simulink model "KUKA_KR10_R1100_ROS"  (R2024a)
settings: Solver=ode15s  StartTime=0.0  StopTime=6  RelTol=1e-9  AbsTol=1e-9  EnableMultiTasking=on
model workspace (MAT data in the model file):
  XSize = 1
values from neighbouring files (symbols this model uses):
  dichte_alu = 2700    [Parameter.m]    (also in workspace_test.mat)
  N = length(accelX)    [pds.m]
undefined symbols (not defined in the file or in its folder): th_J1, th_J2, th_J3, th_J4, th_J5, th_J6, th_transition_factor, X, Y, Z
libraries: sm_lib x70, nesl_utility x30
(part 1 of 3)
settings Model: Creator=beth0005  LastModifiedBy=Johannes
settings SolverCC: AutoScaleAbsTol=off  AlgebraicLoopSolver=TrustRegion
settings DataIOCC: LimitDataPoints=on  MaxDataPoints=10000
settings OptimizationCC: LifeSpan=inf
settings DebuggingCC: UnconnectedInputMsg=warning  UnconnectedOutputMsg=warning  UnconnectedLineMsg=warning  AllowSymbolicDim=off  SFUnexpectedBacktrackingDiag=warning  SFNoUnconditionalDefaultTransitionDiag=warning  SFExecutionAtInitializationDiag=none  ArithmeticOperatorsInVariantConditions=warning
settings ModelReferenceCC: EnableRefExpFcnMdlSchedulingChecks=on
settings SFSimCC: SimUseLocalCustomCode=off  CustomCodeUndefinedFunction=UseInterfaceOnly
settings RTWCC: RTWUseLocalCustomCode=off  GPUComputeCapability=3.5  DLArmComputeVersion=19.05
settings CodeAppCC: StateflowObjectComments=on
settings GRTTargetCC: TargetLangStandard=C89/C90 (ANSI)
settings ConfigComp: CovMetricSettings=dw  CovSaveCumulativeToWorkspaceVar=on  CovSaveSingleToWorkspaceVar=on  CovExternalEMLEnable=off  CovSFcnEnable=off
settings SimscapeCC: SimscapeLogType=all  SimscapeLogSimulationStatistics=on  SimscapeLogDataHistory=10000

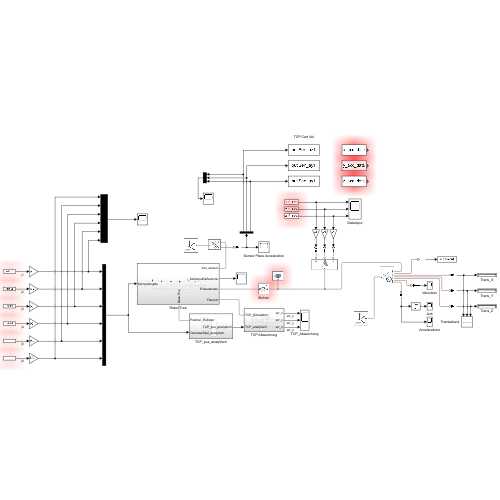
[thumbnail: Simulink's stored preview of the top-level diagram]
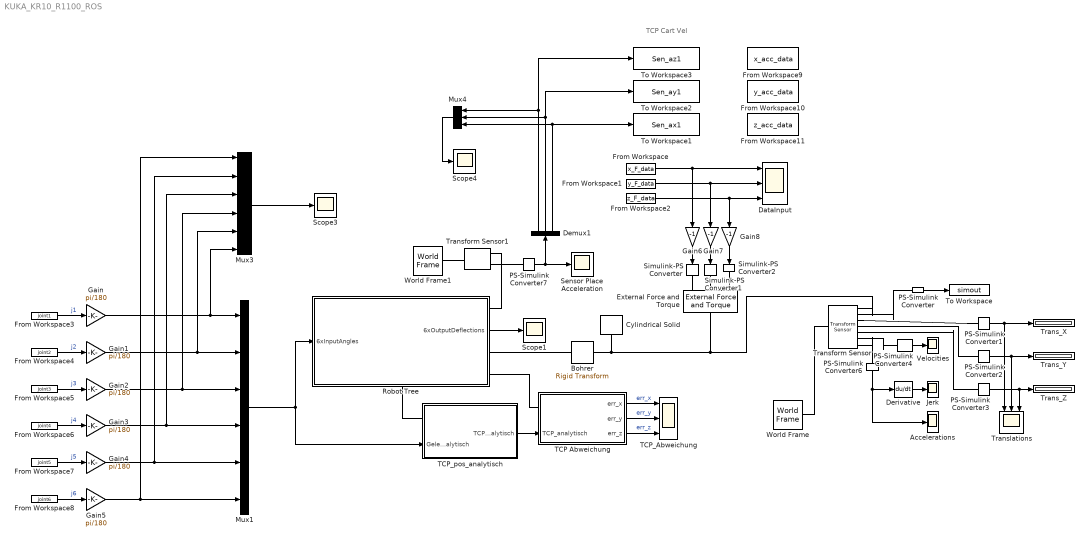
== system KUKA_KR10_R1100_ROS ==
  note: TCP Cart Vel
  Accelerations : Scope
  Bohrer : sm_lib/Frames and Transforms/Rigid Transform  RotationMethod=None  FollAlignAxisA=+X  BaseAlignAxisA=+Y  FollAlignAxisB=+Y  BaseAlignAxisB=+Z  RotationStandardAxis=+Y  RotationAngle=90  RotationAngleUnits=deg  RotationArbitraryAxis=[0 0 1]  RotationSequenceAxes=FollowerAxes  RotationSequence=XYX  RotationSequenceAngles=[0 0 0]  RotationSequenceAnglesUnits=deg  RotationMatrix=[1 0 0; 0 1 0; 0 0 1]  Quaternion=[1 0 0 0]  TranslationMethod=StandardAxis  TranslationCartesianOffset=[0 0 63]  TranslationCartesianOffsetUnits=mm  TranslationStandardAxis=+Z  TranslationStandardOffset=lang_bohrer  TranslationStandardOffsetUnits=mm  TranslationROffset=0  TranslationROffsetUnits=m  TranslationThetaOffset=0  TranslationThetaOffsetUnits=deg  TranslationZOffset=0  TranslationZOffsetUnits=m
  Cylindrical Solid : sm_lib/Body Elements/Cylindrical Solid  CylinderRadius=4  CylinderRadiusUnits=mm  CylinderLength=63  CylinderLengthUnits=mm  ExportEntireGeometry=off  InertiaType=CalculateFromGeometry  BasedOnType=Density  Density=dichte_alu  DensityUnits=kg/m^3  Mass=1  MassUnits=kg  CenterOfMass=[0 0 0]  CenterOfMassUnits=m  MomentsOfInertia=[1 1 1]  MomentsOfInertiaUnits=kg*m^2  ProductsOfInertia=[0 0 0]  ProductsOfInertiaUnits=kg*m^2  GraphicType=FromGeometry  MarkerShape=Sphere  MarkerSize=10  GraphicVisPropType=SimpleVisualProperties  GraphicDiffuseColor=[0.5 0.5 0.5]  GraphicOpacity=1  GraphicSpecularColor=[0.5 0.5 0.5 1.0]  GraphicAmbientColor=[0.15 0.15 0.15 1.0]  GraphicEmissiveColor=[0.0 0.0 0.0 1.0]  GraphicShininess=75  DoExposeReferenceFrame=off  SerializedFrames=<Frames><Frame><Id>Frame1</Id><Value><Name>F1</Name><Origin><Source>GeometricFeature</Source><FeatureName>top surface</FeatureName></Origin><PrimaryAxis><DefinedDirection>+Z</DefinedDirection><Source>ReferenceFrame</Source><SourceDirection>+Z</SourceDirection><FeatureName></FeatureName></PrimaryAxis><SecondaryAxis><DefinedDirection>+X</DefinedDirection><Source>ReferenceFrame</Source><SourceDirection>+X</SourceDirection><FeatureName></FeatureName></SecondaryAxis></Value></Frame></Frames>
  DataInput : Scope  NumInputPorts=3
  Demux1 : Demux  Outputs=3
  Derivative : Derivative
  External Force and Torque : sm_lib/Forces and Torques/External Force and Torque  EnableForceX=on  EnableForceY=on  EnableForceZ=on  EnableForce=off  ForceResolutionFrame=AttachedFrame  EnableTorqueX=off  EnableTorqueY=off  EnableTorqueZ=off  EnableTorque=off  TorqueResolutionFrame=AttachedFrame
  From Workspace : FromWorkspace  VariableName=x_F_data  SampleTime=-1
  From Workspace1 : FromWorkspace  VariableName=y_F_data  SampleTime=-1
  From Workspace10 : FromWorkspace  VariableName=y_acc_data  SampleTime=-1
  From Workspace11 : FromWorkspace  VariableName=z_acc_data  SampleTime=-1
  From Workspace2 : FromWorkspace  VariableName=z_F_data  SampleTime=-1
  From Workspace3 : FromWorkspace  VariableName=joint1  SampleTime=-1
  From Workspace4 : FromWorkspace  VariableName=joint2  SampleTime=-1
  From Workspace5 : FromWorkspace  VariableName=joint3  SampleTime=-1
  From Workspace6 : FromWorkspace  VariableName=joint4  SampleTime=-1
  From Workspace7 : FromWorkspace  VariableName=joint5  SampleTime=-1
  From Workspace8 : FromWorkspace  VariableName=joint6  SampleTime=-1
  From Workspace9 : FromWorkspace  VariableName=x_acc_data  SampleTime=-1
  Gain{,1..5} (6 alike) : Gain  Gain=pi/180
  Gain6 : Gain  Gain=-1
  Gain7 : Gain  Gain=-1
  Gain8 : Gain  Gain=-1
  Jerk : Scope
  Mux1 : Mux  Inputs=6
  Mux3 : Mux  Inputs=6
  Mux4 : Mux  Inputs=3
  PS-Simulink Converter{,1..4,6..7} (7 alike) : nesl_utility/PS-Simulink Converter  PhysicalDomain=network_engine_domain  SubClassName=ps_output  LeftPortType=input  RightPortType=output  PseudoPeriodic=off  Frequencies=[]  VectorFormat=inherit  Unit=inherit  AffineConversion=off
  Robot Tree : Subsystem
      settings: PortSchema="{\"entries\":[{\"content\":{\"sides\":[{\"content\":{\"connectorIds\":[\"In1\"]},\"type\":\"ConnectorPlacement.EquallySpacedRectSide\",\"uuid\":\"83afddbe-1d35-4f48-9dd2-c5eddaf741d9\"},{\"content\":{\"connectorIds\":[\"RConn1\",\"Out1\",\"RConn2\",\"RConn3\"],\"side\":\"RIGHT\"},\"type\":\"ConnectorPlacement.EquallySpacedRectSide\",\"uuid\":\"b2a35604-11db-400a-b921-df56b5b1bdc7\"},{\"content\":{\"side\":\"TOP\"},\"type\":\"ConnectorPlacement.EquallySpacedRectSide\",\"uuid\":\"d988bacb-7459-4110-a132-4d0586d8e44f\"},{\"content\":{\"connectorIds\":[\"RConn4\"],\"side\":\"BOTTOM\"},\"type\":\"ConnectorPlacement.EquallySpacedRectSide\",\"uuid\":\"784d5e4a-8f9a-40d1-a5c6-3fcb642770f1\"}]},\"type\":\"ConnectorPlacement.EquallySpacedConnector\",\"uuid\":\"99878518-e7fe-4a6a-9eb0-094d259cda0e\"}],\"packageUris\":[\"http://schema.mathworks.com/mf0/Connector/R2020b\"],\"version\":\"1.0\"}"
  Scope1 : Scope
  Scope3 : Scope
  Scope4 : Scope
  Sensor Place Acceleration : Scope
  Simulink-PS Converter : nesl_utility/Simulink-PS Converter  PhysicalDomain=network_engine_domain  SubClassName=ps_input  LeftPortType=input  RightPortType=output  PseudoPeriodic=off  Frequencies=[]  NoiseDistribution=none  NoiseParameters=[]  Unit=1  AffineConversion=off  FilteringAndDerivatives=filter  SimscapeFilterOrder=2  InputFilterTimeConstant=0.0001  UdotUserProvided=0
  Simulink-PS Converter1 : nesl_utility/Simulink-PS Converter  PhysicalDomain=network_engine_domain  SubClassName=ps_input  LeftPortType=input  RightPortType=output  PseudoPeriodic=off  Frequencies=[]  NoiseDistribution=none  NoiseParameters=[]  Unit=1  AffineConversion=off  FilteringAndDerivatives=filter  SimscapeFilterOrder=2  InputFilterTimeConstant=0.0001  UdotUserProvided=0
  Simulink-PS Converter2 : nesl_utility/Simulink-PS Converter  PhysicalDomain=network_engine_domain  SubClassName=ps_input  LeftPortType=input  RightPortType=output  PseudoPeriodic=off  Frequencies=[]  NoiseDistribution=none  NoiseParameters=[]  Unit=1  AffineConversion=off  FilteringAndDerivatives=filter  SimscapeFilterOrder=2  InputFilterTimeConstant=0.0001  UdotUserProvided=0
  TCP Abweichung : Subsystem
      settings: PortSchema="{\"entries\":[{\"content\":{\"sides\":[{\"content\":{\"connectorIds\":[\"LConn1\",\"In1\"]},\"type\":\"ConnectorPlacement.EquallySpacedRectSide\",\"uuid\":\"8fbb3f34-d7d1-4090-9281-a387436a6191\"},{\"content\":{\"connectorIds\":[\"Out1\",\"Out2\",\"Out3\"],\"side\":\"RIGHT\"},\"type\":\"ConnectorPlacement.EquallySpacedRectSide\",\"uuid\":\"2461bf91-e690-4063-84b2-ad7cc9454b37\"},{\"content\":{\"side\":\"TOP\"},\"type\":\"ConnectorPlacement.EquallySpacedRectSide\",\"uuid\":\"0fbb9cfb-49b2-42f2-b0a5-a9e967349aea\"}]},\"type\":\"ConnectorPlacement.EquallySpacedConnector\",\"uuid\":\"5e1e4f46-aaa2-4a76-a14e-db38171314b7\"}],\"packageUris\":[\"http://schema.mathworks.com/mf0/Connector/R2020b\"],\"version\":\"1.0\"}"
  TCP_Abweichung : Scope  NumInputPorts=3
  TCP_pos_analytisch : Subsystem
      settings: PortSchema="{\"entries\":[{\"content\":{\"sides\":[{\"content\":{\"connectorIds\":[\"LConn1\",\"In1\"]},\"type\":\"ConnectorPlacement.EquallySpacedRectSide\",\"uuid\":\"538ee7b4-053d-4344-bb82-6fadd6800804\"},{\"content\":{\"connectorIds\":[\"Out1\"],\"side\":\"RIGHT\"},\"type\":\"ConnectorPlacement.EquallySpacedRectSide\",\"uuid\":\"6da0b3fa-3dd3-4693-bc25-55cdb306fc09\"},{\"content\":{\"side\":\"TOP\"},\"type\":\"ConnectorPlacement.EquallySpacedRectSide\",\"uuid\":\"c57a0aac-3147-45b1-888e-d3700a099c5d\"}]},\"type\":\"ConnectorPlacement.EquallySpacedConnector\",\"uuid\":\"ef060d6a-5fd8-4986-b270-7bf484a81e58\"}],\"packageUris\":[\"http://schema.mathworks.com/mf0/Connector/R2020b\"],\"version\":\"1.0\"}"
  To Workspace : ToWorkspace  VariableName=simout  SaveFormat=Structure  SampleTime=-1
  To Workspace1 : ToWorkspace  VariableName=Sen_ax1  SaveFormat=Timeseries  SampleTime=-1
  To Workspace2 : ToWorkspace  VariableName=Sen_ay1  SaveFormat=Timeseries  SampleTime=-1
  To Workspace3 : ToWorkspace  VariableName=Sen_az1  SaveFormat=Timeseries  SampleTime=-1
  Trans_X : Display
  Trans_Y : Display
  Trans_Z : Display
  Transform Sensor : sm_lib/Frames and Transforms/Transform Sensor  MeasurementFrame=World  RotationSequence=XYX  SenseAngle=off  SenseAxis=off  SenseQ=off  SenseR=on  SenseRotationSequence=off  SenseOmegaX=off  SenseOmegaY=off  SenseOmegaZ=off  SenseOmega=off  SenseQDot=off  SenseRDot=off  SenseRotationSequenceDot=off  SenseAlphaX=off  SenseAlphaY=off  SenseAlphaZ=off  SenseAlpha=off  SenseQDDot=off  SenseRDDot=off  SenseX=on  SenseY=on  SenseZ=on  SenseXYZ=off  SenseRad=off  SenseAzim=off  SenseDist=off  SenseInc=off  SenseXDot=off  SenseYDot=off  SenseZDot=off  SenseXYZDot=on  SenseRadDot=off  SenseAzimDot=off  SenseDistDot=off  SenseIncDot=off  SenseXDDot=off  SenseYDDot=off  SenseZDDot=off  SenseXYZDDot=on  SenseRadDDot=off  SenseAzimDDot=off  SenseDistDDot=off  SenseIncDDot=off
  Transform Sensor1 : sm_lib/Frames and Transforms/Transform Sensor  MeasurementFrame=World  RotationSequence=XYX  SenseAngle=off  SenseAxis=off  SenseQ=off  SenseR=off  SenseRotationSequence=off  SenseOmegaX=off  SenseOmegaY=off  SenseOmegaZ=off  SenseOmega=off  SenseQDot=off  SenseRDot=off  SenseRotationSequenceDot=off  SenseAlphaX=off  SenseAlphaY=off  SenseAlphaZ=off  SenseAlpha=off  SenseQDDot=off  SenseRDDot=off  SenseX=off  SenseY=off  SenseZ=off  SenseXYZ=off  SenseRad=off  SenseAzim=off  SenseDist=off  SenseInc=off  SenseXDot=off  SenseYDot=off  SenseZDot=off  SenseXYZDot=off  SenseRadDot=off  SenseAzimDot=off  SenseDistDot=off  SenseIncDot=off  SenseXDDot=off  SenseYDDot=off  SenseZDDot=off  SenseXYZDDot=on  SenseRadDDot=off  SenseAzimDDot=off  SenseDistDDot=off  SenseIncDDot=off
  Translations : Scope  NumInputPorts=3
  Velocities : Scope
  World Frame : sm_lib/Frames and Transforms/World Frame
  World Frame1 : sm_lib/Frames and Transforms/World Frame
  wires:
  From Workspace3/1 -> Gain/1  "j1"
  From Workspace5/1 -> Gain2/1  "j3"
  From Workspace8/1 -> Gain5/1  "j6"
  From Workspace7/1 -> Gain4/1  "j5"
  From Workspace6/1 -> Gain3/1  "j4"
  From Workspace4/1 -> Gain1/1  "j2"
  Robot Tree/1(6xOutputDeflections) -> Scope1/1
  PS-Simulink Converter/1 -> To Workspace/1
  TCP Abweichung/2(err_y) -> TCP_Abweichung/2  "err_y"
  PS-Simulink Converter2/1 -> Trans_Y/1, Translations/2
  TCP Abweichung/3(err_z) -> TCP_Abweichung/3  "err_z"
  TCP Abweichung/1(err_x) -> TCP_Abweichung/1  "err_x"
  TCP_pos_analytisch/1(TCP_pos_analytisch) -> TCP Abweichung/1(TCP_analytisch)
  PS-Simulink Converter1/1 -> Trans_X/1, Translations/1
  PS-Simulink Converter3/1 -> Trans_Z/1, Translations/3
  Mux1/1 -> TCP_pos_analytisch/1(Gelenkwinkel_analytisch), Robot Tree/1(6xInputAngles)
  PS-Simulink Converter4/1 -> Velocities/1
  PS-Simulink Converter6/1 -> Accelerations/1, Derivative/1
  Derivative/1 -> Jerk/1
  From Workspace2/1 -> Gain8/1, DataInput/3
  From Workspace1/1 -> DataInput/2, Gain7/1
  From Workspace/1 -> DataInput/1, Gain6/1
  Gain4/1 -> Mux1/5, Mux3/2
  Gain1/1 -> Mux1/2, Mux3/5
  Gain2/1 -> Mux1/3, Mux3/4
  Gain3/1 -> Mux1/4, Mux3/3
  Gain/1 -> Mux1/1, Mux3/6
  Mux3/1 -> Scope3/1
  Gain5/1 -> Mux1/6, Mux3/1
  Gain6/1 -> Simulink-PS Converter/1
  Gain7/1 -> Simulink-PS Converter1/1
  Gain8/1 -> Simulink-PS Converter2/1
  Demux1/2 -> To Workspace2/1, Mux4/2
  Mux4/1 -> Scope4/1
  Demux1/3 -> To Workspace1/1, Mux4/3
  Demux1/1 -> To Workspace3/1, Mux4/1
  PS-Simulink Converter7/1 -> Sensor Place Acceleration/1, Demux1/1
  connections:
  PS-Simulink Converter3/LConn1 -- Transform Sensor/RConn5
  Transform Sensor/RConn6 -- PS-Simulink Converter4/LConn1
  PS-Simulink Converter1/LConn1 -- Transform Sensor/RConn3
  TCP Abweichung/LConn1 -- Robot Tree/RConn3
  PS-Simulink Converter2/LConn1 -- Transform Sensor/RConn4
  TCP_pos_analytisch/LConn1 -- Robot Tree/RConn4
  World Frame/RConn1 -- Transform Sensor/LConn1
  PS-Simulink Converter/LConn1 -- Transform Sensor/RConn2
  External Force and Torque/RConn1 -- Cylindrical Solid/LConn1 -- Bohrer/RConn1 -- Transform Sensor/RConn1
  Simulink-PS Converter/RConn1 -- External Force and Torque/LConn1
  Simulink-PS Converter2/RConn1 -- External Force and Torque/LConn3
  External Force and Torque/LConn2 -- Simulink-PS Converter1/RConn1
  PS-Simulink Converter6/LConn1 -- Transform Sensor/RConn7
  Bohrer/LConn1 -- Robot Tree/RConn2
  World Frame1/RConn1 -- Transform Sensor1/LConn1
  Robot Tree/RConn1 -- Transform Sensor1/RConn1
  PS-Simulink Converter7/LConn1 -- Transform Sensor1/RConn2
